simulink model "sensorMCUSlugsMKII"  (Simulink 6.6)
settings: Solver=FixedStepDiscrete  StartTime=0.0  StopTime=10.0  FixedStep=0.01  RelTol=1e-3
InitFcn:
  | mcuInit
values from neighbouring files (symbols this model uses):
  T = 0.01    [initGPS.m]    (also in mcuInit.m)
undefined symbols (not defined in the file or in its folder): baroMeanTemp, baroOffset, baroScale, baroTempK, baseHeight, baseTemp, cubeAccelGain, cubeGyroGain, gaind, getCubeData, getGpsMainData, getMag, hil_getEuler, hil_getRates, hil_getRawRead, hil_getVned, hil_getXYZ, hilRead, lapseRate, logData, magMeanTemp, magOffset, magScale, magTempK, pitotOffset, pitotScale, polesd, powerOffset, powerScale, protParseDecode, sensorMCUInit, spiSend, tempOffset, tempScale, u1, u2, updateAirData, updateAttitude, updateBias, updateDiagnosticFl, updateDiagnosticSh, updateLoadData, updatePilotConsole, updatePosition, updateRawADCData, updateTimeStamp, y1, zerosd
libraries: dsPICdrivers x37, simulink x3, aerolibconvert2 x1
(part 1 of 2)
settings Model: Creator=ASL_Lab  LastModifiedBy=Administrator  BufferReuse=off  ProdHWDeviceType=16-bit Generic
settings OptimizationCC: BlockReduction=off  InlineParams=on  OptimizeBlockIOStorage=off  BufferReuse=off  ExpressionFolding=off  LocalBlockOutputs=off  EfficientFloat2IntCast=on  OptimizeModelRefInitCode=on  LifeSpan=1
settings HardwareCC: ProdBitPerInt=16  ProdEndianess=LittleEndian  ProdWordSize=16  ProdHWDeviceType=16-bit Generic  TargetHWDeviceType=32-bit Generic
settings RTWCC: SystemTargetFile=dspic.tlc  TemplateMakefile=dspic_pic30_gcc.tmf  PostCodeGenCommand=dsPIC_Compile()  Description=Embedded Target for Microchip dsPIC (real-time)  GenerateReport=on  ProcessScript=dspic_make_rtw_hook  CustomHeaderCode="#include \"apDefinitions.h\""  IncludeHyperlinkInReport=on  LaunchReport=on
settings RTWCC: CustomSource=|
  | clib\circBuffer.c
  | clib\sbrk.c
  | clib\gps.c
  | clib\dataLogger.c
  | clib\interProcCommMaster.c
  | clib\conversions.c
  | clib\apUtils.c
  | clib\protDecoder.c
  | clib\DEE.c
  | clib\DEES.s
  | clib\magneto.c
  | clib\adisCube.c
settings CodeAppCC: IgnoreCustomStorageClasses=off
settings STFCustomTargetCC: TargetFcnLib=ansi_tfl_tmw.mat  GenFloatMathFcnCalls=ANSI_C  ModelReferenceCompliant=off  IncludeMdlTerminateFcn=off  CombineOutputUpdateFcns=on  SuppressErrorStatus=on  ERTCustomFileBanners=on  SupportContinuousTime=off  SupportNonInlinedSFcns=off  SystemTargetFile=dspic.tlc
settings ERTTargetCC: TargetFcnLib=ansi_tfl_tmw.mat  GenFloatMathFcnCalls=ANSI_C  ModelReferenceCompliant=off  IncludeMdlTerminateFcn=off  SuppressErrorStatus=on  ModelStepFunctionPrototypeControlCompliant=off  ExtModeMexFile=noextcomm  InlinedParameterPlacement=NonHierarchical  ERTSrcFileBannerTemplate=dsPIC_code_template.cgt  ERTHdrFileBannerTemplate=dsPIC_code_template.cgt  ERTDataSrcFileTemplate=dsPIC_code_template.cgt  ERTDataHdrFileTemplate=dsPIC_code_template.cgt  ERTCustomFileTemplate=dsPIC_main.tlc
settings CustomProperty: DataType=string  Value=C:\PROGRA~1\MATLAB\R2007a\rtw\bin\win32\gmake

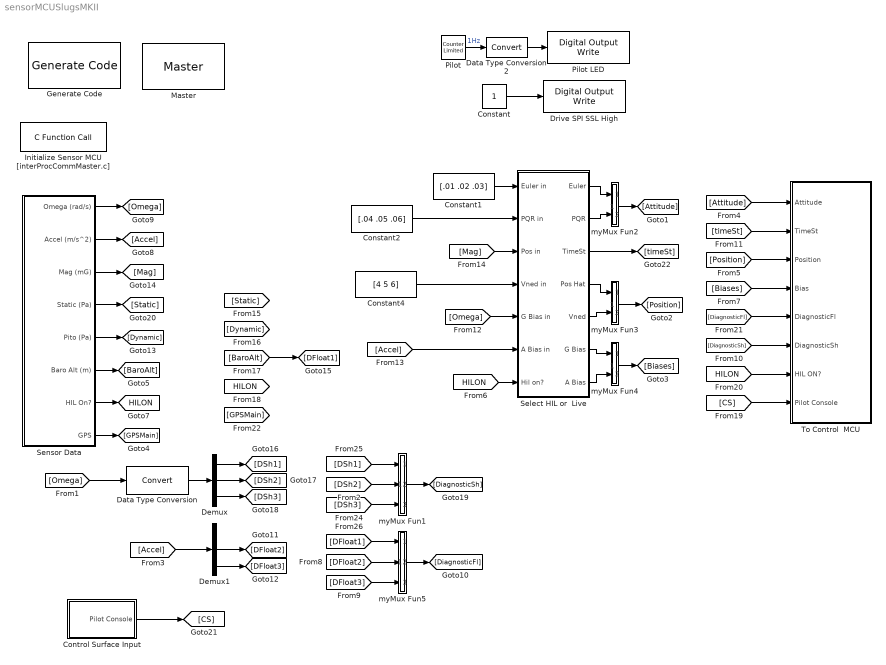
== system sensorMCUSlugsMKII ==
  Constant : Constant  OutDataTypeMode=boolean
  Constant1 : Constant  Value=[.01 .02 .03]  OutDataTypeMode=single
  Constant2 : Constant  Value=[.04 .05 .06]  OutDataTypeMode=single
  Constant4 : Constant  Value=[4 5 6]  OutDataTypeMode=single
  Control Surface Input : Subsystem
  Data Type Conversion : DataTypeConversion  OutDataTypeMode=int16
  Data Type Conversion2 : DataTypeConversion  OutDataTypeMode=boolean
  Demux : Demux  Outputs=3
  Demux1 : Demux  Outputs=3
  Drive SPI SSL High : dsPICdrivers/Digital I//O/Digital Output Write  Tag=dsPIC_Digital_Output  Priority=5  PORT=B  Pin=[ 2]  Simultaneous=off  OrderingInOutPopup=None
  Generate Code : dsPICdrivers/Simulink Configuration/Generate Code
  Initialize Sensor MCU [interProcCommMaster.c] : dsPICdrivers/OTHERS/C Function Call  Tag=dsPIC_dsPIC_CFunctionCall  fctName='sensorMCUInit'  INPUT_SIZE=1  INPUT1=--  INPUT2=--  INPUT3=--  OUTPUT_SIZE=1  OUTPUT1=--  SampleTime=inf  InputType=[ ]  OutputType=[ ]  FctDeclaration=extern void sensorMCUInit();  FctCall=sensorMCUInit();  OrderingInOutPopup=None
  Master : dsPICdrivers/Master  Tag=dsPIC_MASTER  Priority=1  TimeStepType=Timer1  picType=33fJ256MC710  fcy=40000000  Quartz_33f=12e6  PLLActive_33f=on  fcyDesired_33f=40e6  tmr1="[8  49999  0]"  tmr1Info="Time Step : 0.01  ;   Error : 0%  PR1=49999"  tmr2345="[8  0  0  0  0  0  0  0]"  tmr2345cfg=[-1 -1 -1 -1 -1 -1 -1 -1]  IOautoConf=on  typePort="[ 0   0   0   0   0   0   0   0   0   0   0   0   0   0   9   0  10  10  10   0   0   0  10   0   8   8   8   8   0   0   0   0   0   0   0   0   0   0   0   0   0   0   0   0   0   0   0   0   0   0   9   0   0   0   0   0   0   6   6   6   6   0   0   6   0   0   0   0   0   0   0   0   0   0   0   0   0   0   0   0   0   0   0   0   0   0   0   0   0   0   0   0   0   0   0   0   0   0   0   0   0   0   0   0   0   0   0   0   0   0   0   0 ]"  TRIS="[ 65535  65464  65535  65535  65535  65535  65535 ]"  ADPCFG=71  MasterBusyPort=B1  MasterOverloadPort=B6  FOSC=External Clock  ClockSwitchMonitor=Both disabled  TempProtection_33f=TEMP_ON  FPBOR=<empty>  PWRT=64ms  MCLR=<empty>  PowerSave=off  OverrideFcy=off  NewFcy=1e6  PR2345="[65535  65535  65535  65535  65535  65535  65535  65535]"
  Pilot : simulink/Sources/Counter Limited  SystemSampleTime=-1  uplimit=1  tsamp=1.0
  Pilot LED : dsPICdrivers/Digital I//O/Digital Output Write  Tag=dsPIC_Digital_Output  Priority=5  PORT=B  Pin=[0]  Simultaneous=off  OrderingInOutPopup=None
  Select HIL or  Live : Subsystem
  Sensor Data : Subsystem
  To Control  MCU : Subsystem
  myMux Fun1 : Stateflow chart
  myMux Fun2 : Stateflow chart
  myMux Fun3 : Stateflow chart
  myMux Fun4 : Stateflow chart
  myMux Fun5 : Stateflow chart
  tag scope: HILON=global
  wires:
  Pilot/1 -> Data Type Conversion2/1  "1Hz"
  Data Type Conversion2/1 -> Pilot LED/1
  Constant/1 -> Drive SPI SSL High/1
  myMux Fun2/1(y) -> [Attitude]
  myMux Fun3/1(y) -> [Position]
  myMux Fun4/1(y) -> [Biases]
  Demux/1 -> [DSh1]
  Demux/2 -> [DSh2]
  Demux/3 -> [DSh3]
  Control Surface Input/1(Pilot Console) -> [CS]
  [Position] -> To Control  MCU/3(Position)
  [Biases] -> To Control  MCU/4(Bias)
  [DiagnosticFl] -> To Control  MCU/5(DiagnosticFl)
  [HILON] -> To Control  MCU/7(HIL ON?)
  [CS] -> To Control  MCU/8(Pilot Console)
  [Attitude] -> To Control  MCU/1(Attitude)
  Select HIL or  Live/1(Euler) -> myMux Fun2/1(u1)
  Select HIL or  Live/2(PQR) -> myMux Fun2/2(u2)
  Select HIL or  Live/3(TimeSt) -> [timeSt]
  Select HIL or  Live/4(Pos Hat) -> myMux Fun3/1(u1)
  Select HIL or  Live/5(Vned) -> myMux Fun3/2(u2)
  Select HIL or  Live/6(G Bias) -> myMux Fun4/1(u1)
  Select HIL or  Live/7(A Bias) -> myMux Fun4/2(u2)
  [DSh1] -> myMux Fun1/1(u1)
  [DSh2] -> myMux Fun1/2(u2)
  [DSh3] -> myMux Fun1/3(u3)
  [DFloat1] -> myMux Fun5/1(u1)
  [DFloat2] -> myMux Fun5/2(u2)
  [DFloat3] -> myMux Fun5/3(u3)
  myMux Fun1/1(y) -> [DiagnosticSh]
  myMux Fun5/1(y) -> [DiagnosticFl]
  [DiagnosticSh] -> To Control  MCU/6(DiagnosticSh)
  [timeSt] -> To Control  MCU/2(TimeSt)
  Sensor Data/2(Accel (m/s^2)) -> [Accel]
  Sensor Data/1(Omega (rad/s)) -> [Omega]
  Sensor Data/3(Mag (mG)) -> [Mag]
  Sensor Data/4(Static (Pa)) -> [Static]
  Sensor Data/5(Pito (Pa)) -> [Dynamic]
  Sensor Data/6(Baro Alt (m)) -> [BaroAlt]
  Sensor Data/7(HIL On?) -> [HILON]
  Sensor Data/8(GPS) -> [GPSMain]
  Demux1/2 -> [DFloat2]
  Demux1/3 -> [DFloat3]
  Data Type Conversion/1 -> Demux/1
  [Omega] -> Data Type Conversion/1
  [Accel] -> Demux1/1
  [HILON] -> Select HIL or  Live/7(Hil on?)
  Constant1/1 -> Select HIL or  Live/1(Euler in)
  Constant2/1 -> Select HIL or  Live/2(PQR in)
  [Mag] -> Select HIL or  Live/3(Pos in)
  Constant4/1 -> Select HIL or  Live/4(Vned in)
  [Omega] -> Select HIL or  Live/5(G Bias in)
  [Accel] -> Select HIL or  Live/6(A Bias in)
  [BaroAlt] -> [DFloat1]

== system sensorMCUSlugsMKII/Control Surface Input ==
  Input Capture : dsPICdrivers/Peripheral I//O/Input Capture  Tag=dsPIC_PWM_IC  Priority=5  IntPriority=6  Channel=[ 2 3 4 5 8]  Channel_UP_Down_Periode="[1  1  1  1  1]"  MaxChannel="[0.0025      0.0025      0.0025      0.0025      0.0025]"  SafeMarge="[10  10  10  10  10]"  MaxName=' IC2max , IC3max , IC4max , IC5max , IC8max '  Precision="[13.7469      13.7469      13.7469      13.7469      13.7469]"  Timer="[2  2  2  2  2]"  ChangeDetected="[0  0  0  0  0]"  ChangeDetectedPortRef=3  SampleTime=.01  Status=OK
  myMux Fun5 : Stateflow chart
  Pilot Console : Outport
  wires:
  myMux Fun5/1(y) -> Pilot Console/1
  Input Capture/1 -> myMux Fun5/1(u1)
  Input Capture/2 -> myMux Fun5/2(u2)
  Input Capture/3 -> myMux Fun5/3(u3)
  Input Capture/4 -> myMux Fun5/4(u4)
  Input Capture/5 -> myMux Fun5/5(u5)

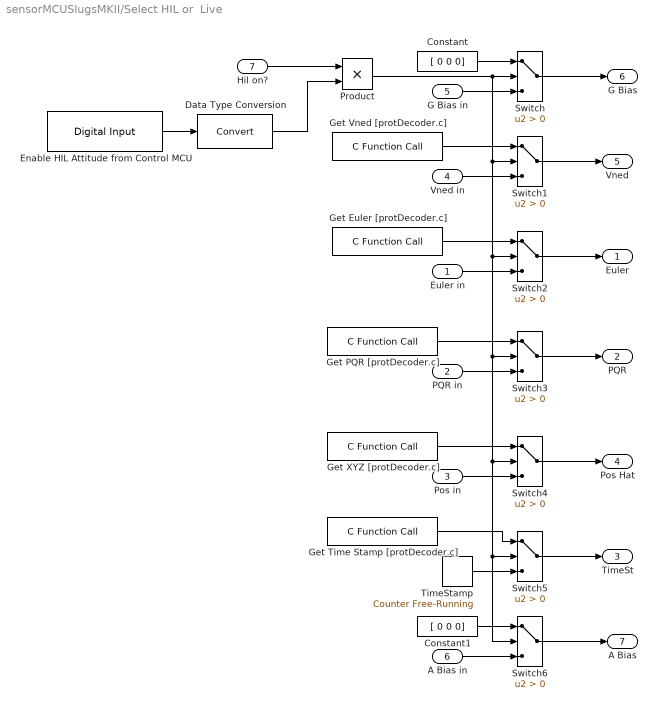
== system sensorMCUSlugsMKII/Select HIL or  Live ==
  Euler in : Inport
  PQR in : Inport  Port=2
  Pos in : Inport  Port=3
  Vned in : Inport  Port=4
  G Bias in : Inport  Port=5
  A Bias in : Inport  Port=6
  Hil on? : Inport  Port=7
  Constant : Constant  Value=[ 0 0 0]  OutDataTypeMode=single
  Constant1 : Constant  Value=[ 0 0 0]  OutDataTypeMode=single
  Data Type Conversion : DataTypeConversion  OutDataTypeMode=uint8
  Enable HIL Attitude from Control MCU : dsPICdrivers/Digital I//O/Digital Input  Tag=dsPIC_Digital_Input  PORT=A  Pin=[14]  SampleTime=.01  OrderingInOutPopup=None
  Get Euler [protDecoder.c] : dsPICdrivers/OTHERS/C Function Call  Tag=dsPIC_dsPIC_CFunctionCall  fctName='hil_getEuler'  INPUT_SIZE=1  INPUT1=--  INPUT2=--  INPUT3=--  OUTPUT_SIZE=3  OUTPUT1=real32  SampleTime=.01  InputType=[ ]  OutputType=[ 7 ]  FctDeclaration=extern void hil_getEuler(real32_T* y1);  FctCall=hil_getEuler(*%y1);  OrderingInOutPopup=None
  Get PQR [protDecoder.c] : dsPICdrivers/OTHERS/C Function Call  Tag=dsPIC_dsPIC_CFunctionCall  fctName='hil_getRates'  INPUT_SIZE=1  INPUT1=--  INPUT2=--  INPUT3=--  OUTPUT_SIZE=3  OUTPUT1=real32  SampleTime=.01  InputType=[ ]  OutputType=[ 7 ]  FctDeclaration=extern void hil_getRates(real32_T* y1);  FctCall=hil_getRates(*%y1);  OrderingInOutPopup=None
  Get Time Stamp [protDecoder.c] : dsPICdrivers/OTHERS/C Function Call  Tag=dsPIC_dsPIC_CFunctionCall  fctName='hil_getTs'  INPUT_SIZE=1  INPUT1=--  INPUT2=--  INPUT3=--  OUTPUT_SIZE=1  OUTPUT1=uint16  SampleTime=.01  InputType=[ ]  OutputType=[ 4 ]  FctDeclaration=extern uint16_T hil_getTs();  FctCall=%y1 = hil_getTs();  OrderingInOutPopup=None
  Get Vned [protDecoder.c] : dsPICdrivers/OTHERS/C Function Call  Tag=dsPIC_dsPIC_CFunctionCall  fctName='hil_getVned'  INPUT_SIZE=1  INPUT1=--  INPUT2=--  INPUT3=--  OUTPUT_SIZE=3  OUTPUT1=real32  SampleTime=.01  InputType=[ ]  OutputType=[ 7 ]  FctDeclaration=extern void hil_getVned(real32_T* y1);  FctCall=hil_getVned(*%y1);  OrderingInOutPopup=None
  Get XYZ [protDecoder.c] : dsPICdrivers/OTHERS/C Function Call  Tag=dsPIC_dsPIC_CFunctionCall  fctName='hil_getXYZ'  INPUT_SIZE=1  INPUT1=--  INPUT2=--  INPUT3=--  OUTPUT_SIZE=3  OUTPUT1=real32  SampleTime=.01  InputType=[ ]  OutputType=[ 7 ]  FctDeclaration=extern void hil_getXYZ(real32_T* y1);  FctCall=hil_getXYZ(*%y1);  OrderingInOutPopup=None
  Product : Product  OutDataTypeMode=uint8  RndMeth=Zero
  Switch{,1..6} (7 alike) : Switch  Criteria=u2 > Threshold
  TimeStamp : simulink/Sources/Counter Free-Running  SystemSampleTime=-1  NumBits=16  tsamp=.01
  Euler : Outport
  PQR : Outport  Port=2
  TimeSt : Outport  Port=3
  Pos Hat : Outport  Port=4
  Vned : Outport  Port=5
  G Bias : Outport  Port=6
  A Bias : Outport  Port=7
  wires:
  Switch/1 -> G Bias/1
  Constant/1 -> Switch/1
  Product/1 -> Switch/2, Switch1/2, Switch2/2, Switch3/2, Switch4/2, Switch5/2, Switch6/2
  G Bias in/1 -> Switch/3
  Switch1/1 -> Vned/1
  Get Vned [protDecoder.c]/1 -> Switch1/1
  Vned in/1 -> Switch1/3
  Get Euler [protDecoder.c]/1 -> Switch2/1
  Euler in/1 -> Switch2/3
  Switch2/1 -> Euler/1
  Get PQR [protDecoder.c]/1 -> Switch3/1
  PQR in/1 -> Switch3/3
  Switch3/1 -> PQR/1
  Get XYZ [protDecoder.c]/1 -> Switch4/1
  Pos in/1 -> Switch4/3
  Switch4/1 -> Pos Hat/1
  TimeStamp/1 -> Switch5/3
  Get Time Stamp [protDecoder.c]/1 -> Switch5/1
  Enable HIL Attitude from Control MCU/1 -> Data Type Conversion/1
  Hil on?/1 -> Product/1
  Data Type Conversion/1 -> Product/2
  Switch5/1 -> TimeSt/1
  Switch6/1 -> A Bias/1
  Constant1/1 -> Switch6/1
  A Bias in/1 -> Switch6/3

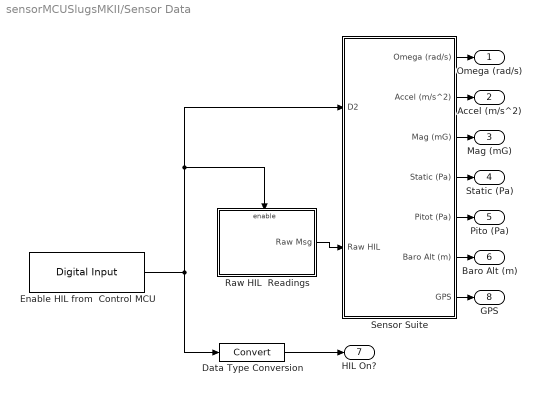
== system sensorMCUSlugsMKII/Sensor Data ==
  Data Type Conversion : DataTypeConversion  OutDataTypeMode=uint8  SampleTime=0.01
  Enable HIL from  Control MCU : dsPICdrivers/Digital I//O/Digital Input  Tag=dsPIC_Digital_Input  PORT=D  Pin=[2]  SampleTime=.01  OrderingInOutPopup=None
  Raw HIL  Readings : Subsystem
  Sensor Suite : Subsystem
  Omega (rad/s) : Outport
  Accel (m/s^2) : Outport  Port=2
  Mag (mG) : Outport  Port=3
  Static (Pa) : Outport  Port=4
  Pito (Pa) : Outport  Port=5
  Baro Alt (m) : Outport  Port=6
  HIL On? : Outport  Port=7
  GPS : Outport  Port=8
  wires:
  Raw HIL  Readings/1(Raw Msg) -> Sensor Suite/2(Raw HIL)
  Enable HIL from  Control MCU/1 -> Raw HIL  Readings/Enable, Sensor Suite/1(D2), Data Type Conversion/1
  Data Type Conversion/1 -> HIL On?/1
  Sensor Suite/1(Omega (rad/s)) -> Omega (rad/s)/1
  Sensor Suite/2(Accel (m/s^2)) -> Accel (m/s^2)/1
  Sensor Suite/3(Mag (mG)) -> Mag (mG)/1
  Sensor Suite/4(Static (Pa)) -> Static (Pa)/1
  Sensor Suite/5(Pitot (Pa)) -> Pito (Pa)/1
  Sensor Suite/6(Baro Alt (m)) -> Baro Alt (m)/1
  Sensor Suite/7(GPS) -> GPS/1

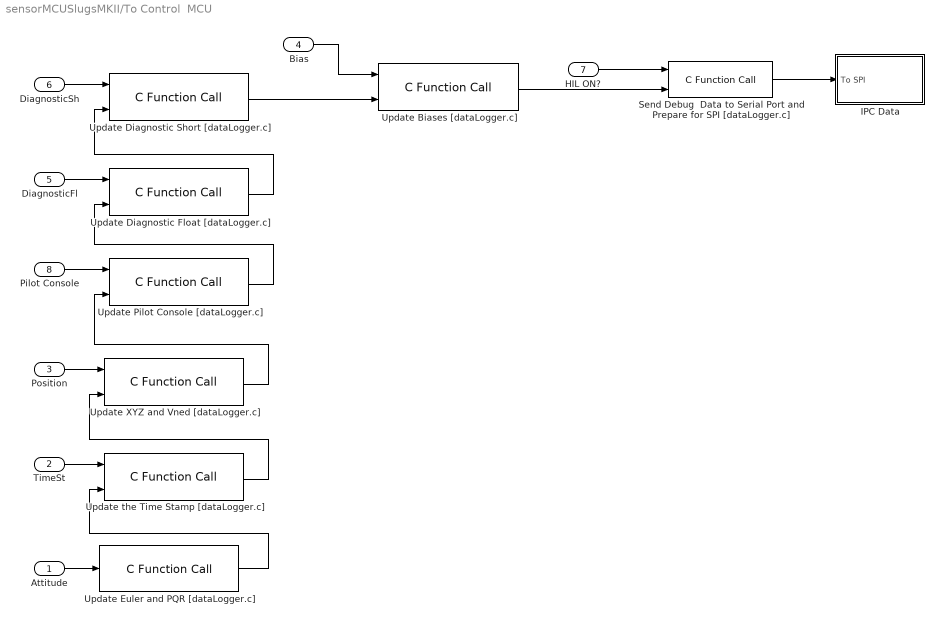
== system sensorMCUSlugsMKII/To Control  MCU ==
  Attitude : Inport
  TimeSt : Inport  Port=2
  Position : Inport  Port=3
  Bias : Inport  Port=4
  DiagnosticFl : Inport  Port=5
  DiagnosticSh : Inport  Port=6
  HIL ON? : Inport  Port=7
  Pilot Console : Inport  Port=8
  IPC Data : Subsystem
  Send Debug  Data to Serial Port and Prepare for SPI [dataLogger.c] : dsPICdrivers/OTHERS/C Function Call  Tag=dsPIC_dsPIC_CFunctionCall  fctName='logData'  INPUT_SIZE=1  INPUT1=uint8  INPUT2=--  INPUT3=--  OUTPUT_SIZE=104  OUTPUT1=uint8  SampleTime=-1  InputType=[ 2 ]  OutputType=[ 2 ]  FctDeclaration=extern void logData(uint8_T u1,uint8_T* y1);  FctCall=logData(%u1, *%y1);  OrderingInOutPopup=Input
  Update Biases [dataLogger.c] : dsPICdrivers/OTHERS/C Function Call  Tag=dsPIC_dsPIC_CFunctionCall  fctName='updateBias'  INPUT_SIZE=6  INPUT1=real32  INPUT2=--  INPUT3=--  OUTPUT_SIZE=1  OUTPUT1=--  SampleTime=.01  InputType=[ 7 ]  OutputType=[ ]  FctDeclaration=extern void updateBias(real32_T* u1);  FctCall=updateBias(*%u1);  OrderingInOutPopup=Input & Output
  Update Diagnostic Float [dataLogger.c] : dsPICdrivers/OTHERS/C Function Call  Tag=dsPIC_dsPIC_CFunctionCall  fctName='updateDiagnosticFl'  INPUT_SIZE=3  INPUT1=real32  INPUT2=--  INPUT3=--  OUTPUT_SIZE=1  OUTPUT1=--  SampleTime=.01  InputType=[ 7 ]  OutputType=[ ]  FctDeclaration=extern void updateDiagnosticFl(real32_T* u1);  FctCall=updateDiagnosticFl(*%u1);  OrderingInOutPopup=Input & Output
  Update Diagnostic Short [dataLogger.c] : dsPICdrivers/OTHERS/C Function Call  Tag=dsPIC_dsPIC_CFunctionCall  fctName='updateDiagnosticSh'  INPUT_SIZE=3  INPUT1=int16  INPUT2=--  INPUT3=--  OUTPUT_SIZE=1  OUTPUT1=--  SampleTime=.01  InputType=[ 3 ]  OutputType=[ ]  FctDeclaration=extern void updateDiagnosticSh(int16_T* u1);  FctCall=updateDiagnosticSh(*%u1);  OrderingInOutPopup=Input & Output
  Update Euler and PQR [dataLogger.c] : dsPICdrivers/OTHERS/C Function Call  Tag=dsPIC_dsPIC_CFunctionCall  fctName='updateAttitude'  INPUT_SIZE=6  INPUT1=real32  INPUT2=--  INPUT3=--  OUTPUT_SIZE=1  OUTPUT1=--  SampleTime=.01  InputType=[ 7 ]  OutputType=[ ]  FctDeclaration=extern void updateAttitude(real32_T* u1);  FctCall=updateAttitude(*%u1);  OrderingInOutPopup=Output
  Update Pilot Console [dataLogger.c] : dsPICdrivers/OTHERS/C Function Call  Tag=dsPIC_dsPIC_CFunctionCall  fctName='updatePilotConsole'  INPUT_SIZE=5  INPUT1=uint16  INPUT2=--  INPUT3=--  OUTPUT_SIZE=1  OUTPUT1=--  SampleTime=.01  InputType=[ 4 ]  OutputType=[ ]  FctDeclaration=extern void updatePilotConsole(uint16_T* u1);  FctCall=updatePilotConsole(*%u1);  OrderingInOutPopup=Input & Output
  Update XYZ and Vned [dataLogger.c] : dsPICdrivers/OTHERS/C Function Call  Tag=dsPIC_dsPIC_CFunctionCall  fctName='updatePosition'  INPUT_SIZE=6  INPUT1=real32  INPUT2=--  INPUT3=--  OUTPUT_SIZE=1  OUTPUT1=--  SampleTime=.01  InputType=[ 7 ]  OutputType=[ ]  FctDeclaration=extern void updatePosition(real32_T* u1);  FctCall=updatePosition(*%u1);  OrderingInOutPopup=Input & Output
  Update the Time Stamp [dataLogger.c] : dsPICdrivers/OTHERS/C Function Call  Tag=dsPIC_dsPIC_CFunctionCall  fctName='updateTimeStamp'  INPUT_SIZE=1  INPUT1=uint16  INPUT2=--  INPUT3=--  OUTPUT_SIZE=1  OUTPUT1=--  SampleTime=.01  InputType=[ 4 ]  OutputType=[ ]  FctDeclaration=extern void updateTimeStamp(uint16_T u1);  FctCall=updateTimeStamp(%u1);  OrderingInOutPopup=Input & Output
  wires:
  Send Debug  Data to Serial Port and Prepare for SPI [dataLogger.c]/1 -> IPC Data/1(To SPI)
  HIL ON?/1 -> Send Debug  Data to Serial Port and Prepare for SPI [dataLogger.c]/1
  Attitude/1 -> Update Euler and PQR [dataLogger.c]/1
  Update Euler and PQR [dataLogger.c]/1 -> Update the Time Stamp [dataLogger.c]/2
  TimeSt/1 -> Update the Time Stamp [dataLogger.c]/1
  Update the Time Stamp [dataLogger.c]/1 -> Update XYZ and Vned [dataLogger.c]/2
  Position/1 -> Update XYZ and Vned [dataLogger.c]/1
  Update XYZ and Vned [dataLogger.c]/1 -> Update Pilot Console [dataLogger.c]/2
  Pilot Console/1 -> Update Pilot Console [dataLogger.c]/1
  DiagnosticFl/1 -> Update Diagnostic Float [dataLogger.c]/1
  Update Pilot Console [dataLogger.c]/1 -> Update Diagnostic Float [dataLogger.c]/2
  Update Diagnostic Float [dataLogger.c]/1 -> Update Diagnostic Short [dataLogger.c]/2
  DiagnosticSh/1 -> Update Diagnostic Short [dataLogger.c]/1
  Update Biases [dataLogger.c]/1 -> Send Debug  Data to Serial Port and Prepare for SPI [dataLogger.c]/2
  Update Diagnostic Short [dataLogger.c]/1 -> Update Biases [dataLogger.c]/2
  Bias/1 -> Update Biases [dataLogger.c]/1

== system sensorMCUSlugsMKII/Sensor Data/Raw HIL  Readings ==
  Enable : EnablePort
  GetRawMsg [protDecoder.c] : dsPICdrivers/OTHERS/C Function Call  Tag=dsPIC_dsPIC_CFunctionCall  fctName='hil_getRawRead'  INPUT_SIZE=1  INPUT1=--  INPUT2=--  INPUT3=--  OUTPUT_SIZE=13  OUTPUT1=int16  SampleTime=0.01  InputType=[ ]  OutputType=[ 3 ]  FctDeclaration=extern void hil_getRawRead(int16_T* y1);  FctCall=hil_getRawRead(*%y1);  OrderingInOutPopup=Input
  Parser/Decoder [protDecoder.c] : dsPICdrivers/OTHERS/C Function Call  Tag=dsPIC_dsPIC_CFunctionCall  fctName='protParseDecode'  INPUT_SIZE=103  INPUT1=uint8  INPUT2=--  INPUT3=--  OUTPUT_SIZE=1  OUTPUT1=--  SampleTime=-1  InputType=[ 2 ]  OutputType=[ ]  FctDeclaration=extern void protParseDecode(uint8_T* u1);  FctCall=protParseDecode(*%u1);  OrderingInOutPopup=Output
  Read Data from HIL3 [dataLogger.c] : dsPICdrivers/OTHERS/C Function Call  Tag=dsPIC_dsPIC_CFunctionCall  fctName='hilRead'  INPUT_SIZE=1  INPUT1=--  INPUT2=--  INPUT3=--  OUTPUT_SIZE=103  OUTPUT1=uint8  SampleTime=0.01  InputType=[ ]  OutputType=[ 2 ]  FctDeclaration=extern void hilRead(uint8_T* y1);  FctCall=hilRead(*%y1);  OrderingInOutPopup=None
  Raw Msg : Outport
  wires:
  GetRawMsg [protDecoder.c]/1 -> Raw Msg/1
  Read Data from HIL3 [dataLogger.c]/1 -> Parser/Decoder [protDecoder.c]/1
  Parser/Decoder [protDecoder.c]/1 -> GetRawMsg [protDecoder.c]/1

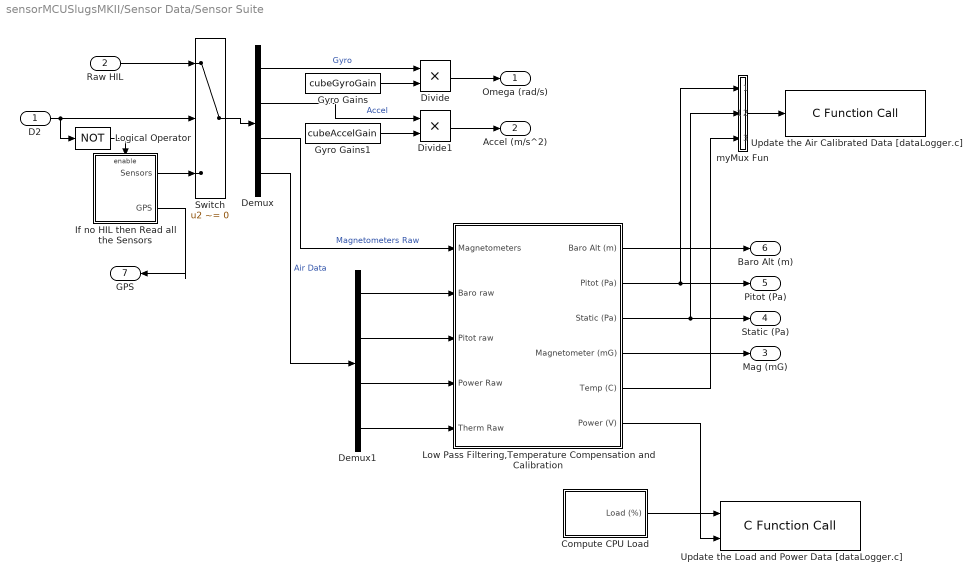
== system sensorMCUSlugsMKII/Sensor Data/Sensor Suite ==
  D2 : Inport
  Raw HIL : Inport  Port=2
  Compute CPU Load : Subsystem
  Demux : Demux  Outputs=[3 3 3 4]
  Demux1 : Demux
  Divide : Product  OutDataTypeMode=single  OutScaling=2^-10
  Divide1 : Product  OutDataTypeMode=single  OutScaling=2^-10
  Gyro Gains : Constant  Value=cubeGyroGain  OutDataTypeMode=single
  Gyro Gains1 : Constant  Value=cubeAccelGain  OutDataTypeMode=single
  If no HIL then Read all the Sensors : Subsystem
  Logical Operator : Logic  Operator=NOT  AllPortsSameDT=off  OutDataTypeMode=Boolean
  Low Pass Filtering,Temperature Compensation and Calibration : Subsystem
  Switch : Switch  Criteria=u2 ~= 0  SampleTime=0.01
  Update the Air Calibrated Data [dataLogger.c] : dsPICdrivers/OTHERS/C Function Call  Tag=dsPIC_dsPIC_CFunctionCall  fctName='updateAirData'  INPUT_SIZE=3  INPUT1=real32  INPUT2=--  INPUT3=--  OUTPUT_SIZE=1  OUTPUT1=--  SampleTime=.01  InputType=[ 7 ]  OutputType=[ ]  FctDeclaration=extern void updateAirData(real32_T* u1);  FctCall=updateAirData(*%u1);  OrderingInOutPopup=None
  Update the Load and Power Data [dataLogger.c] : dsPICdrivers/OTHERS/C Function Call  Tag=dsPIC_dsPIC_CFunctionCall  fctName='updateLoadData'  INPUT_SIZE=1  INPUT1=uint8  INPUT2=uint16  INPUT3=--  OUTPUT_SIZE=1  OUTPUT1=--  SampleTime=.01  InputType=[ 2 4 ]  OutputType=[ ]  FctDeclaration=extern void updateLoadData(uint8_T u1, uint16_T u2);  FctCall=updateLoadData(%u1, %u2);  OrderingInOutPopup=None
  myMux Fun : Stateflow chart
  Omega (rad/s) : Outport
  Accel (m/s^2) : Outport  Port=2
  Mag (mG) : Outport  Port=3
  Static (Pa) : Outport  Port=4
  Pitot (Pa) : Outport  Port=5
  Baro Alt (m) : Outport  Port=6
  GPS : Outport  Orientation=left  Port=7
  wires:
  Switch/1 -> Demux/1
  D2/1 -> Switch/2, Logical Operator/1
  If no HIL then Read all the Sensors/1(Sensors) -> Switch/3
  Logical Operator/1 -> If no HIL then Read all the Sensors/Enable
  Raw HIL/1 -> Switch/1
  Low Pass Filtering,Temperature Compensation and Calibration/1(Baro Alt (m)) -> Baro Alt (m)/1
  Gyro Gains/1 -> Divide/2
  Demux/1 -> Divide/1  "Gyro"
  Divide/1 -> Omega (rad/s)/1
  Gyro Gains1/1 -> Divide1/2
  Demux/2 -> Divide1/1  "Accel"
  Divide1/1 -> Accel (m/s^2)/1
  Demux/4 -> Demux1/1  "Air Data"
  Demux1/1 -> Low Pass Filtering,Temperature Compensation and Calibration/2(Baro raw)
  Demux1/2 -> Low Pass Filtering,Temperature Compensation and Calibration/3(Pitot raw)
  Demux1/4 -> Low Pass Filtering,Temperature Compensation and Calibration/5(Therm Raw)
  Demux/3 -> Low Pass Filtering,Temperature Compensation and Calibration/1(Magnetometers)  "Magnetometers Raw"
  Demux1/3 -> Low Pass Filtering,Temperature Compensation and Calibration/4(Power Raw)
  Low Pass Filtering,Temperature Compensation and Calibration/2(Pitot (Pa)) -> Pitot (Pa)/1, myMux Fun/1(u1)
  Low Pass Filtering,Temperature Compensation and Calibration/3(Static (Pa)) -> Static (Pa)/1, myMux Fun/2(u2)
  Low Pass Filtering,Temperature Compensation and Calibration/4(Magnetometer (mG)) -> Mag (mG)/1
  myMux Fun/1(y) -> Update the Air Calibrated Data [dataLogger.c]/1
  Low Pass Filtering,Temperature Compensation and Calibration/5(Temp (C)) -> myMux Fun/3(u3)
  Compute CPU Load/1(Load (%)) -> Update the Load and Power Data [dataLogger.c]/1
  Low Pass Filtering,Temperature Compensation and Calibration/6(Power (V)) -> Update the Load and Power Data [dataLogger.c]/2
  If no HIL then Read all the Sensors/2(GPS) -> GPS/1

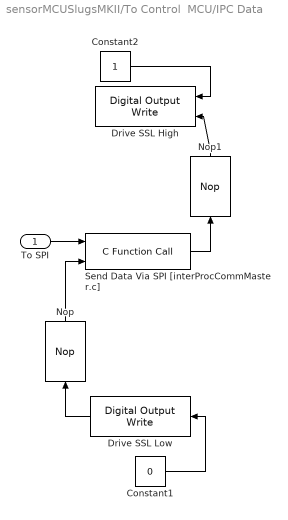
== system sensorMCUSlugsMKII/To Control  MCU/IPC Data ==
  To SPI : Inport
  Constant1 : Constant  Value=0  OutDataTypeMode=boolean  SampleTime=.01
  Constant2 : Constant  OutDataTypeMode=boolean
  Drive SSL High : dsPICdrivers/Digital I//O/Digital Output Write  Tag=dsPIC_Digital_Output  Orientation=left  Priority=5  PORT=B  Pin=[ 2]  Simultaneous=off  OrderingInOutPopup=Input
  Drive SSL Low : dsPICdrivers/Digital I//O/Digital Output Write  Tag=dsPIC_Digital_Output  Orientation=left  Priority=5  PORT=B  Pin=[ 2]  Simultaneous=off  OrderingInOutPopup=Output
  Nop : dsPICdrivers/OTHERS/Nop  Tag=dsPIC_Reset  Orientation=up  NbrNop=10
  Nop1 : dsPICdrivers/OTHERS/Nop  Tag=dsPIC_Reset  Orientation=up  NbrNop=10
  Send Data Via SPI [interProcCommMaster.c] : dsPICdrivers/OTHERS/C Function Call  Tag=dsPIC_dsPIC_CFunctionCall  fctName='spiSend'  INPUT_SIZE=104  INPUT1=uint8  INPUT2=--  INPUT3=--  OUTPUT_SIZE=1  OUTPUT1=--  SampleTime=-1  InputType=[ 2 ]  OutputType=[ ]  FctDeclaration=extern void spiSend(uint8_T* u1);  FctCall=spiSend(*%u1);  OrderingInOutPopup=Input & Output
  wires:
  Constant1/1 -> Drive SSL Low/1
  Drive SSL Low/1 -> Nop/1
  Constant2/1 -> Drive SSL High/1
  Send Data Via SPI [interProcCommMaster.c]/1 -> Nop1/1
  To SPI/1 -> Send Data Via SPI [interProcCommMaster.c]/1
  Nop/1 -> Send Data Via SPI [interProcCommMaster.c]/2
  Nop1/1 -> Drive SSL High/2

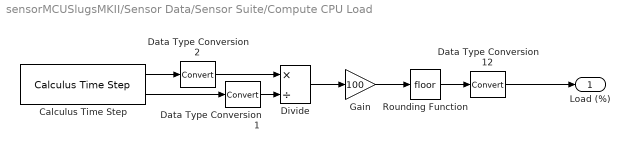
== system sensorMCUSlugsMKII/Sensor Data/Sensor Suite/Compute CPU Load ==
  Calculus Time Step : dsPICdrivers/OTHERS/Calculus Time Step  Tag=dsPIC_CalculusTimeStep  SampleTime=0.01  PR1chk=on
  Data Type Conversion1 : DataTypeConversion  OutDataTypeMode=single
  Data Type Conversion12 : DataTypeConversion  OutDataTypeMode=uint8
  Data Type Conversion2 : DataTypeConversion  OutDataTypeMode=single
  Divide : Product  Inputs=*/  OutDataTypeMode=double  OutScaling=2^-10
  Gain : Gain  Gain=100
  Rounding Function : Rounding
  Load (%) : Outport
  wires:
  Calculus Time Step/1 -> Data Type Conversion2/1
  Calculus Time Step/2 -> Data Type Conversion1/1
  Divide/1 -> Gain/1
  Rounding Function/1 -> Data Type Conversion12/1
  Data Type Conversion1/1 -> Divide/2
  Data Type Conversion2/1 -> Divide/1
  Data Type Conversion12/1 -> Load (%)/1
  Gain/1 -> Rounding Function/1

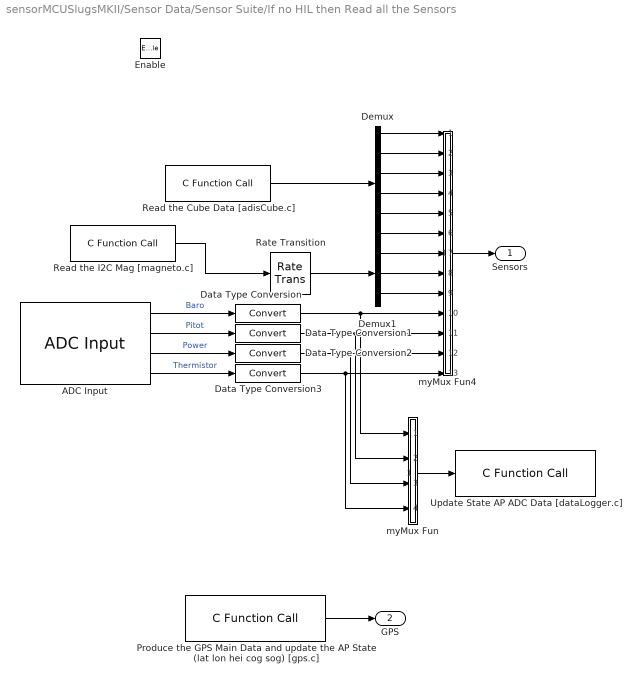
== system sensorMCUSlugsMKII/Sensor Data/Sensor Suite/If no HIL then Read all the Sensors ==
  Enable : EnablePort
  ADC Input : dsPICdrivers/Peripheral I//O/ADC Input  Tag=dsPIC_ADC  Priority=5  ADC_TYPE=12 bits  ADC_MODE=Continuous sampling & get last channel value  NbrSampleStep=1  VoltRefpopup="AVdd  -  AVss"  OutFormatBitspopup=0000 dddd dddd dddd : Integer  InterruptPriority=6  ANCHANNELS=[8 9 10 11]  MaxName=ANmax = 4095  Rin=200  ADCS=53  SAMC=1  Temperature=25  DMAChannel=1  SampleTime=.01  Status="OK  |  Tsmp=6.750e-007 |  T/Channel=1.012e-005 |  Tall=4.050e-005"  SSRC=auto convert
  Data Type Conversion{,1..3} (4 alike) : DataTypeConversion  OutDataTypeMode=int16
  Demux : Demux  Outputs=6
  Demux1 : Demux  Outputs=3
  Produce the GPS Main Data and update the AP State (lat lon hei cog sog) [gps.c] : dsPICdrivers/OTHERS/C Function Call  Tag=dsPIC_dsPIC_CFunctionCall  fctName='getGpsMainData'  INPUT_SIZE=1  INPUT1=--  INPUT2=--  INPUT3=--  OUTPUT_SIZE=5  OUTPUT1=real32  SampleTime=.01  InputType=[ ]  OutputType=[ 7 ]  FctDeclaration=extern void getGpsMainData(real32_T* y1);  FctCall=getGpsMainData(*%y1);  OrderingInOutPopup=None
  Rate Transition : RateTransition  OutPortSampleTime=0.01
  Read the Cube Data [adisCube.c] : dsPICdrivers/OTHERS/C Function Call  Tag=dsPIC_dsPIC_CFunctionCall  fctName='getCubeData'  INPUT_SIZE=1  INPUT1=--  INPUT2=--  INPUT3=--  OUTPUT_SIZE=6  OUTPUT1=int16  SampleTime=.01  InputType=[ ]  OutputType=[ 3 ]  FctDeclaration=extern void getCubeData(int16_T* y1);  FctCall=getCubeData(*%y1);  OrderingInOutPopup=None
  Read the I2C Mag [magneto.c] : dsPICdrivers/OTHERS/C Function Call  Tag=dsPIC_dsPIC_CFunctionCall  fctName='getMag'  INPUT_SIZE=1  INPUT1=--  INPUT2=--  INPUT3=--  OUTPUT_SIZE=3  OUTPUT1=int16  SampleTime=.01  InputType=[ ]  OutputType=[ 3 ]  FctDeclaration=extern void getMag(int16_T* y1);  FctCall=getMag(*%y1);  OrderingInOutPopup=None
  Update State AP ADC Data [dataLogger.c] : dsPICdrivers/OTHERS/C Function Call  Tag=dsPIC_dsPIC_CFunctionCall  fctName='updateRawADCData'  INPUT_SIZE=4  INPUT1=int16  INPUT2=--  INPUT3=--  OUTPUT_SIZE=1  OUTPUT1=--  SampleTime=.01  InputType=[ 3 ]  OutputType=[ ]  FctDeclaration=extern void updateRawADCData(int16_T* u1);  FctCall=updateRawADCData(*%u1);  OrderingInOutPopup=None
  myMux Fun : Stateflow chart
  myMux Fun4 : Stateflow chart
  Sensors : Outport
  GPS : Outport  Port=2
  wires:
  myMux Fun4/1(y) -> Sensors/1
  Read the Cube Data [adisCube.c]/1 -> Demux/1
  Read the I2C Mag [magneto.c]/1 -> Rate Transition/1
  Demux/1 -> myMux Fun4/1(u1)
  Demux/2 -> myMux Fun4/2(u2)
  Demux/3 -> myMux Fun4/3(u3)
  Demux/4 -> myMux Fun4/4(u4)
  Demux/5 -> myMux Fun4/5(u5)
  Demux/6 -> myMux Fun4/6(u6)
  Demux1/1 -> myMux Fun4/7(u7)
  Demux1/2 -> myMux Fun4/8(u8)
  Demux1/3 -> myMux Fun4/9(u9)
  ADC Input/1 -> Data Type Conversion/1  "Baro"
  ADC Input/2 -> Data Type Conversion1/1  "Pitot"
  ADC Input/3 -> Data Type Conversion2/1  "Power"
  ADC Input/4 -> Data Type Conversion3/1  "Thermistor"
  myMux Fun/1(y) -> Update State AP ADC Data [dataLogger.c]/1
  Rate Transition/1 -> Demux1/1
  Data Type Conversion/1 -> myMux Fun4/10(u10), myMux Fun/1(u1)
  Data Type Conversion1/1 -> myMux Fun4/11(u11), myMux Fun/2(u2)
  Data Type Conversion2/1 -> myMux Fun4/12(u12), myMux Fun/3(u3)
  Data Type Conversion3/1 -> myMux Fun4/13(u13), myMux Fun/4(u4)
  Produce the GPS Main Data and update the AP State (lat lon hei cog sog) [gps.c]/1 -> GPS/1

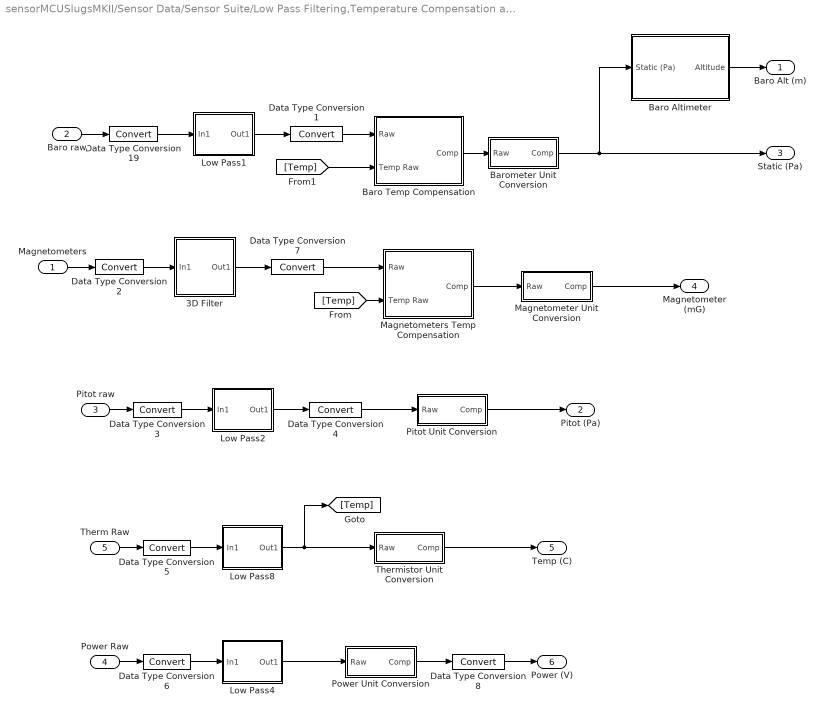
== system sensorMCUSlugsMKII/Sensor Data/Sensor Suite/Low Pass Filtering,Temperature Compensation and Calibration ==
  Magnetometers : Inport
  Baro raw : Inport  Port=2
  Pitot raw : Inport  Port=3
  Power Raw : Inport  Port=4
  Therm Raw : Inport  Port=5
  3D Filter : Subsystem  AncestorBlock=SLUGS_Library/Singnal Routing & Conditioning/3D Filter  RTWFcnName=TustinFilter3D  mask{zval=[], pval=-150, kval=150, TSample=0.01}
      mask prompts: zval "Zeros"; pval "Poles"; kval "Gains"; TSample "Sample Time"
      settings: RTWFcnNameOpts=User specified  RTWFileNameOpts=Use function name
      mask Display:
      | droots(zval,pval,kval)
      | port_label('input',1,'3D')
  Baro Altimeter : Subsystem
  Baro Temp Compensation : Subsystem  mask{alpha=baroTempK, tempMean=baroMeanTemp}
      mask prompts: alpha "Tempearature Coeficient (K_t)"; tempMean "Calibration Temperature Mean (T_avg)"
      mask help:
      | This block implements a temperature compensation. It implmements the following equation:
      |
      | M_tc = M_raw - K_t(T - T_avg)
  Barometer Unit Conversion : Subsystem  mask{bias=baroOffset, gains=baroScale}
      mask prompts: bias "Initial Bias"; gains "Initial Gains"
      mask help: Convert Analog readings to units
  Data Type Conversion1 : DataTypeConversion  OutDataTypeMode=single
  Data Type Conversion{2..3,5..6,19} (5 alike) : DataTypeConversion  OutDataTypeMode=double
  Data Type Conversion4 : DataTypeConversion  OutDataTypeMode=single
  Data Type Conversion7 : DataTypeConversion  OutDataTypeMode=single
  Data Type Conversion8 : DataTypeConversion  OutDataTypeMode=uint16
  Low Pass1 : Subsystem  mask(DiscretizedZeroPole){Zeros=[], Poles=[-30], Gain=30, AbsTol=auto, SampleTime=T, method=tustin, Wc=1}
      mask prompts: Zeros "Zeros (enter in s-main:)"; Poles "Poles (enter in s-domain:)"; Gain "Gain (enter in s-domain:)"; AbsTol "Absolute tolerance:"; SampleTime "Sample time:"; Wc "Critical Frequency (Hz):"
      mask help: Continuous mask uses c2d to transform parameters onto the Discrete Zero-Pole block inside.
      mask init:
      | st=SampleTime;
      | if length(st)>1
      |     st=SampleTime(1);
      | end
      | if(st>0)
      |     [zerosd,polesd,gaind] = sldiscutil('disczpk', {st,method,Wc,Zeros,Poles,Gain});
      | end	
      | s = get_param(gcb,'maskvalues');
      | zeross = s{1};
      | poless = s{2};
      | gainss = s{3};
      | %zerosc = eval(zeross);
      | %polesc = eval(poless);
      | %gainsc = eval(gainss);
      | sldiscutil('initzpkmask', st);
      | if(st==0)
      | set_param([gcb '/Zero Pole'], 'AbsoluteTolerance', AbsTol);
      | end
      mask StyleString: edit,edit,edit,edit,edit,popup(zoh|foh|tustin|prewarp|matched),edit
      mask CallbackString: |||||hidecrit|
      mask Display:
      | droots(zeross,poless,gainss)
      | text( 0.5, 1.0, method, 'verticalAlignment','top')
  Low Pass2 : Subsystem  mask(DiscretizedZeroPole){Zeros=[], Poles=[-30], Gain=30, AbsTol=auto, SampleTime=T, method=tustin, Wc=1}
      mask prompts: Zeros "Zeros (enter in s-main:)"; Poles "Poles (enter in s-domain:)"; Gain "Gain (enter in s-domain:)"; AbsTol "Absolute tolerance:"; SampleTime "Sample time:"; Wc "Critical Frequency (Hz):"
      mask help: Continuous mask uses c2d to transform parameters onto the Discrete Zero-Pole block inside.
      mask init: same as sensorMCUSlugsMKII/Sensor Data/Sensor Suite/Low Pass Filtering,Temperature Compensation and Calibration/Low Pass1
      mask StyleString: edit,edit,edit,edit,edit,popup(zoh|foh|tustin|prewarp|matched),edit
      mask CallbackString: |||||hidecrit|
      mask Display:
      | droots(zeross,poless,gainss)
      | text( 0.5, 1.0, method, 'verticalAlignment','top')
  Low Pass4 : Subsystem  mask(DiscretizedZeroPole){Zeros=[], Poles=[-3], Gain=3, AbsTol=auto, SampleTime=T, method=tustin, Wc=1}
      mask prompts: Zeros "Zeros (enter in s-main:)"; Poles "Poles (enter in s-domain:)"; Gain "Gain (enter in s-domain:)"; AbsTol "Absolute tolerance:"; SampleTime "Sample time:"; Wc "Critical Frequency (Hz):"
      mask help: Continuous mask uses c2d to transform parameters onto the Discrete Zero-Pole block inside.
      mask init: same as sensorMCUSlugsMKII/Sensor Data/Sensor Suite/Low Pass Filtering,Temperature Compensation and Calibration/Low Pass1
      mask StyleString: edit,edit,edit,edit,edit,popup(zoh|foh|tustin|prewarp|matched),edit
      mask CallbackString: |||||hidecrit|
      mask Display:
      | droots(zeross,poless,gainss)
      | text( 0.5, 1.0, method, 'verticalAlignment','top')
  Low Pass8 : Subsystem  mask(DiscretizedZeroPole){Zeros=[], Poles=[-10], Gain=10, AbsTol=auto, SampleTime=T, method=tustin, Wc=1}
      mask prompts: Zeros "Zeros (enter in s-main:)"; Poles "Poles (enter in s-domain:)"; Gain "Gain (enter in s-domain:)"; AbsTol "Absolute tolerance:"; SampleTime "Sample time:"; Wc "Critical Frequency (Hz):"
      mask help: Continuous mask uses c2d to transform parameters onto the Discrete Zero-Pole block inside.
      mask init: same as sensorMCUSlugsMKII/Sensor Data/Sensor Suite/Low Pass Filtering,Temperature Compensation and Calibration/Low Pass1
      mask StyleString: edit,edit,edit,edit,edit,popup(zoh|foh|tustin|prewarp|matched),edit
      mask CallbackString: |||||hidecrit|
      mask Display:
      | droots(zeross,poless,gainss)
      | text( 0.5, 1.0, method, 'verticalAlignment','top')
  Magnetometer Unit Conversion : Subsystem  mask{bias=magOffset, gains=magScale}
      mask prompts: bias "Initial Bias"; gains "Initial Gains"
      mask help: Convert Analog readings to units
  Magnetometers Temp Compensation : Subsystem  mask{alpha=magTempK, tempMean=magMeanTemp}
      mask prompts: alpha "Tempearature Coeficient (K_t)"; tempMean "Calibration Temperature Mean (T_avg)"
      mask help:
      | This block implements a temperature compensation. It implmements the following equation:
      |
      | M_tc = M_raw - K_t(T - T_avg)
  Pitot Unit Conversion : Subsystem  mask{bias=pitotOffset, gains=pitotScale}
      mask prompts: bias "Initial Bias"; gains "Initial Gains"
      mask help: Convert Analog readings to units
  Power Unit Conversion : Subsystem  mask{bias=powerOffset, gains=powerScale}
      mask prompts: bias "Initial Bias"; gains "Initial Gains"
      mask help: Convert Analog readings to units
  Thermistor Unit Conversion : Subsystem  mask{bias=tempOffset, gains=tempScale}
      mask prompts: bias "Initial Bias"; gains "Initial Gains"
      mask help: Convert Analog readings to units
  Baro Alt (m) : Outport
  Pitot (Pa) : Outport  Port=2
  Static (Pa) : Outport  Port=3
  Magnetometer (mG) : Outport  Port=4
  Temp (C) : Outport  Port=5
  Power (V) : Outport  Port=6
  wires:
  Data Type Conversion19/1 -> Low Pass1/1(In1)
  Data Type Conversion3/1 -> Low Pass2/1(In1)
  Low Pass2/1(Out1) -> Data Type Conversion4/1
  Data Type Conversion5/1 -> Low Pass8/1(In1)
  Barometer Unit Conversion/1(Comp) -> Static (Pa)/1, Baro Altimeter/1(Static (Pa))
  Baro raw/1 -> Data Type Conversion19/1
  Pitot raw/1 -> Data Type Conversion3/1
  Therm Raw/1 -> Data Type Conversion5/1
  Baro Temp Compensation/1(Comp) -> Barometer Unit Conversion/1(Raw)
  Data Type Conversion2/1 -> 3D Filter/1(In1)
  3D Filter/1(Out1) -> Data Type Conversion7/1
  Magnetometers/1 -> Data Type Conversion2/1
  Pitot Unit Conversion/1(Comp) -> Pitot (Pa)/1
  Low Pass8/1(Out1) -> [Temp], Thermistor Unit Conversion/1(Raw)
  Data Type Conversion4/1 -> Pitot Unit Conversion/1(Raw)
  Data Type Conversion7/1 -> Magnetometers Temp Compensation/1(Raw)
  Magnetometers Temp Compensation/1(Comp) -> Magnetometer Unit Conversion/1(Raw)
  [Temp] -> Magnetometers Temp Compensation/2(Temp Raw)
  Magnetometer Unit Conversion/1(Comp) -> Magnetometer (mG)/1
  Low Pass1/1(Out1) -> Data Type Conversion1/1
  [Temp] -> Baro Temp Compensation/2(Temp Raw)
  Data Type Conversion1/1 -> Baro Temp Compensation/1(Raw)
  Thermistor Unit Conversion/1(Comp) -> Temp (C)/1
  Data Type Conversion6/1 -> Low Pass4/1(In1)
  Power Raw/1 -> Data Type Conversion6/1
  Low Pass4/1(Out1) -> Power Unit Conversion/1(Raw)
  Power Unit Conversion/1(Comp) -> Data Type Conversion8/1
  Data Type Conversion8/1 -> Power (V)/1
  Baro Altimeter/1(Altitude) -> Baro Alt (m)/1

== system sensorMCUSlugsMKII/Sensor Data/Sensor Suite/Low Pass Filtering,Temperature Compensation and Calibration/3D Filter ==
  In1 : Inport
  Demux : Demux  Outputs=3
  Filter1 : Subsystem  mask(DiscretizedZeroPole){Zeros=zval, Poles=pval, Gain=kval, AbsTol=auto, SampleTime=TSample, method=tustin, Wc=1}
      mask prompts: Zeros "Zeros (enter in s-main:)"; Poles "Poles (enter in s-domain:)"; Gain "Gain (enter in s-domain:)"; AbsTol "Absolute tolerance:"; SampleTime "Sample time:"; Wc "Critical Frequency (Hz):"
      mask help: Continuous mask uses c2d to transform parameters onto the Discrete Zero-Pole block inside.
      mask init: same as sensorMCUSlugsMKII/Sensor Data/Sensor Suite/Low Pass Filtering,Temperature Compensation and Calibration/Low Pass1
      mask StyleString: edit,edit,edit,edit,edit,popup(zoh|foh|tustin|prewarp|matched),edit
      mask CallbackString: |||||hidecrit|
      mask Display:
      | droots(zeross,poless,gainss)
      | text( 0.5, 1.0, method, 'verticalAlignment','top')
  Filter2 : Subsystem  mask(DiscretizedZeroPole){Zeros=zval, Poles=pval, Gain=kval, AbsTol=auto, SampleTime=TSample, method=tustin, Wc=1}
      mask prompts: Zeros "Zeros (enter in s-main:)"; Poles "Poles (enter in s-domain:)"; Gain "Gain (enter in s-domain:)"; AbsTol "Absolute tolerance:"; SampleTime "Sample time:"; Wc "Critical Frequency (Hz):"
      mask help: Continuous mask uses c2d to transform parameters onto the Discrete Zero-Pole block inside.
      mask init: same as sensorMCUSlugsMKII/Sensor Data/Sensor Suite/Low Pass Filtering,Temperature Compensation and Calibration/Low Pass1
      mask StyleString: edit,edit,edit,edit,edit,popup(zoh|foh|tustin|prewarp|matched),edit
      mask CallbackString: |||||hidecrit|
      mask Display:
      | droots(zeross,poless,gainss)
      | text( 0.5, 1.0, method, 'verticalAlignment','top')
  Filter3 : Subsystem  mask(DiscretizedZeroPole){Zeros=zval, Poles=pval, Gain=kval, AbsTol=auto, SampleTime=TSample, method=tustin, Wc=1}
      mask prompts: Zeros "Zeros (enter in s-main:)"; Poles "Poles (enter in s-domain:)"; Gain "Gain (enter in s-domain:)"; AbsTol "Absolute tolerance:"; SampleTime "Sample time:"; Wc "Critical Frequency (Hz):"
      mask help: Continuous mask uses c2d to transform parameters onto the Discrete Zero-Pole block inside.
      mask init: same as sensorMCUSlugsMKII/Sensor Data/Sensor Suite/Low Pass Filtering,Temperature Compensation and Calibration/Low Pass1
      mask StyleString: edit,edit,edit,edit,edit,popup(zoh|foh|tustin|prewarp|matched),edit
      mask CallbackString: |||||hidecrit|
      mask Display:
      | droots(zeross,poless,gainss)
      | text( 0.5, 1.0, method, 'verticalAlignment','top')
  myMux Fun1 : Stateflow chart
  Out1 : Outport
  wires:
  myMux Fun1/1(y) -> Out1/1
  In1/1 -> Demux/1
  Filter3/1(Out1) -> myMux Fun1/3(u3)
  Filter2/1(Out1) -> myMux Fun1/2(u2)
  Filter1/1(Out1) -> myMux Fun1/1(u1)
  Demux/3 -> Filter3/1(In1)
  Demux/2 -> Filter2/1(In1)
  Demux/1 -> Filter1/1(In1)

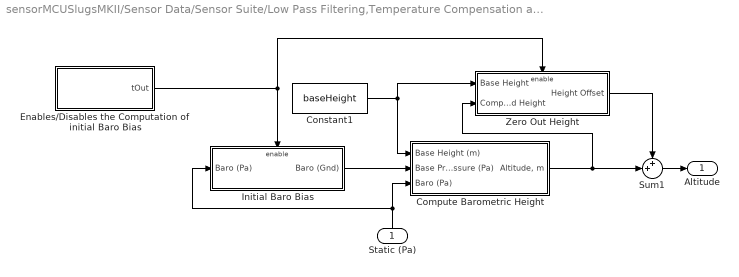
== system sensorMCUSlugsMKII/Sensor Data/Sensor Suite/Low Pass Filtering,Temperature Compensation and Calibration/Baro Altimeter ==
  Static (Pa) : Inport  Orientation=up
  Compute Barometric Height : Subsystem  mask{baseTemp=baseTemp, LapseRate=lapseRate}
      mask prompts: baseTemp "Base Station Temperature (K)"; LapseRate "Lapse Rate (C/ft)"
      mask help:
      | Produces Altitude in meters from Barometric Pressure in Pascals. Altitude is valid from MSL to 6000 ft.
      |
      | The method implemented here was developed by Ren Curry
  Constant1 : Constant  Value=baseHeight  OutDataTypeMode=single
  Enables/Disables the Computation of  initial Baro Bias : Stateflow chart
  Initial Baro Bias : Subsystem  TreatAsAtomicUnit=on
  Sum1 : Sum  Inputs=++|  OutDataTypeMode=single
  Zero Out Height : Subsystem  TreatAsAtomicUnit=on
  Altitude : Outport
  wires:
  Compute Barometric Height/1("Altitude, m") -> Zero Out Height/2(Computed Height), Sum1/2
  Static (Pa)/1 -> Initial Baro Bias/1(Baro (Pa)), Compute Barometric Height/3(Baro (Pa))
  Enables/Disables the Computation of  initial Baro Bias/1(tOut) -> Initial Baro Bias/Enable, Zero Out Height/Enable
  Constant1/1 -> Compute Barometric Height/1(Base Height (m)), Zero Out Height/1(Base Height)
  Initial Baro Bias/1(Baro (Gnd)) -> Compute Barometric Height/2(Base Pressure (Pa))
  Zero Out Height/1(Height Offset) -> Sum1/1
  Sum1/1 -> Altitude/1

== system sensorMCUSlugsMKII/Sensor Data/Sensor Suite/Low Pass Filtering,Temperature Compensation and Calibration/Baro Temp Compensation ==
  Raw : Inport
  Temp Raw : Inport  Port=2
  Divide1 : Product  OutDataTypeMode=single  OutScaling=2^-10
  Mean Temperature for Calibration : Constant  Value=tempMean  OutDataTypeMode=single
  Sum1 : Sum  Inputs=|+-  OutDataTypeMode=single
  Sum2 : Sum  Inputs=|+-  OutDataTypeMode=single
  gains : Constant  Value=alpha  OutDataTypeMode=single
  Comp : Outport
  wires:
  Mean Temperature for Calibration/1 -> Sum1/2
  Raw/1 -> Sum2/1
  Temp Raw/1 -> Sum1/1
  Sum1/1 -> Divide1/2
  gains/1 -> Divide1/1
  Divide1/1 -> Sum2/2
  Sum2/1 -> Comp/1

== system sensorMCUSlugsMKII/Sensor Data/Sensor Suite/Low Pass Filtering,Temperature Compensation and Calibration/Barometer Unit Conversion ==
  Raw : Inport
  Bias : Constant  Value=bias  OutDataTypeMode=single
  Divide : Product  OutDataTypeMode=single  OutScaling=2^-10
  Gains : Constant  Value=gains  OutDataTypeMode=single
  Sum : Sum  Inputs=|++  OutDataTypeMode=single
  Comp : Outport
  wires:
  Bias/1 -> Sum/2
  Raw/1 -> Divide/2
  Gains/1 -> Divide/1
  Divide/1 -> Sum/1
  Sum/1 -> Comp/1

== system sensorMCUSlugsMKII/Sensor Data/Sensor Suite/Low Pass Filtering,Temperature Compensation and Calibration/Low Pass1 ==
  In1 : Inport
  Discrete Zero-Pole : DiscreteZeroPole  Zeros=zerosd  Poles=polesd  Gain=gaind  SampleTime=SampleTime
  Out1 : Outport
  wires:
  In1/1 -> Discrete Zero-Pole/1
  Discrete Zero-Pole/1 -> Out1/1

== system sensorMCUSlugsMKII/Sensor Data/Sensor Suite/Low Pass Filtering,Temperature Compensation and Calibration/Low Pass2 ==
  In1 : Inport
  Discrete Zero-Pole : DiscreteZeroPole  Zeros=zerosd  Poles=polesd  Gain=gaind  SampleTime=SampleTime
  Out1 : Outport
  wires:
  Discrete Zero-Pole/1 -> Out1/1
  In1/1 -> Discrete Zero-Pole/1

== system sensorMCUSlugsMKII/Sensor Data/Sensor Suite/Low Pass Filtering,Temperature Compensation and Calibration/Low Pass4 ==
  In1 : Inport
  Discrete Zero-Pole : DiscreteZeroPole  Zeros=zerosd  Poles=polesd  Gain=gaind  SampleTime=SampleTime
  Out1 : Outport
  wires:
  Discrete Zero-Pole/1 -> Out1/1
  In1/1 -> Discrete Zero-Pole/1

== system sensorMCUSlugsMKII/Sensor Data/Sensor Suite/Low Pass Filtering,Temperature Compensation and Calibration/Low Pass8 ==
  In1 : Inport
  Discrete Zero-Pole : DiscreteZeroPole  Zeros=zerosd  Poles=polesd  Gain=gaind  SampleTime=SampleTime
  Out1 : Outport
  wires:
  In1/1 -> Discrete Zero-Pole/1
  Discrete Zero-Pole/1 -> Out1/1

== system sensorMCUSlugsMKII/Sensor Data/Sensor Suite/Low Pass Filtering,Temperature Compensation and Calibration/Magnetometer Unit Conversion ==
  Raw : Inport
  Bias : Constant  Value=bias  OutDataTypeMode=single
  Divide : Product  OutDataTypeMode=single  OutScaling=2^-10
  Gains : Constant  Value=gains  OutDataTypeMode=single
  Sum : Sum  Inputs=|++  OutDataTypeMode=single
  Comp : Outport
  wires:
  Sum/1 -> Comp/1
  Divide/1 -> Sum/1
  Gains/1 -> Divide/1
  Raw/1 -> Divide/2
  Bias/1 -> Sum/2

== system sensorMCUSlugsMKII/Sensor Data/Sensor Suite/Low Pass Filtering,Temperature Compensation and Calibration/Magnetometers Temp Compensation ==
  Raw : Inport
  Temp Raw : Inport  Port=2
  Divide1 : Product  OutDataTypeMode=single  OutScaling=2^-10
  Mean Temperature for Calibration : Constant  Value=tempMean  OutDataTypeMode=single
  Sum1 : Sum  Inputs=|+-  OutDataTypeMode=single
  Sum2 : Sum  Inputs=|+-  OutDataTypeMode=single
  gains : Constant  Value=alpha  OutDataTypeMode=single
  Comp : Outport
  wires:
  Sum2/1 -> Comp/1
  Divide1/1 -> Sum2/2
  gains/1 -> Divide1/1
  Sum1/1 -> Divide1/2
  Temp Raw/1 -> Sum1/1
  Raw/1 -> Sum2/1
  Mean Temperature for Calibration/1 -> Sum1/2

== system sensorMCUSlugsMKII/Sensor Data/Sensor Suite/Low Pass Filtering,Temperature Compensation and Calibration/Pitot Unit Conversion ==
  Raw : Inport
  Bias : Constant  Value=bias  OutDataTypeMode=single
  Divide : Product  OutDataTypeMode=single  OutScaling=2^-10
  Gains : Constant  Value=gains  OutDataTypeMode=single
  Sum : Sum  Inputs=|++  OutDataTypeMode=single
  Comp : Outport
  wires:
  Bias/1 -> Sum/2
  Raw/1 -> Divide/2
  Gains/1 -> Divide/1
  Divide/1 -> Sum/1
  Sum/1 -> Comp/1

== system sensorMCUSlugsMKII/Sensor Data/Sensor Suite/Low Pass Filtering,Temperature Compensation and Calibration/Power Unit Conversion ==
  Raw : Inport
  Bias : Constant  Value=bias  OutDataTypeMode=single
  Divide : Product  OutDataTypeMode=single  OutScaling=2^-10
  Gains : Constant  Value=gains  OutDataTypeMode=single
  Sum : Sum  Inputs=|++  OutDataTypeMode=single
  Comp : Outport
  wires:
  Bias/1 -> Sum/2
  Raw/1 -> Divide/2
  Gains/1 -> Divide/1
  Divide/1 -> Sum/1
  Sum/1 -> Comp/1

== system sensorMCUSlugsMKII/Sensor Data/Sensor Suite/Low Pass Filtering,Temperature Compensation and Calibration/Thermistor Unit Conversion ==
  Raw : Inport
  Bias : Constant  Value=bias  OutDataTypeMode=single
  Divide : Product  OutDataTypeMode=single  OutScaling=2^-10
  Gains : Constant  Value=gains  OutDataTypeMode=single
  Sum : Sum  Inputs=|++  OutDataTypeMode=single
  Comp : Outport
  wires:
  Sum/1 -> Comp/1
  Divide/1 -> Sum/1
  Gains/1 -> Divide/1
  Raw/1 -> Divide/2
  Bias/1 -> Sum/2

== system sensorMCUSlugsMKII/Sensor Data/Sensor Suite/Low Pass Filtering,Temperature Compensation and Calibration/3D Filter/Filter1 ==
  In1 : Inport
  Discrete Zero-Pole : DiscreteZeroPole  Zeros=zerosd  Poles=polesd  Gain=gaind  SampleTime=SampleTime
  Out1 : Outport
  wires:
  Discrete Zero-Pole/1 -> Out1/1
  In1/1 -> Discrete Zero-Pole/1

== system sensorMCUSlugsMKII/Sensor Data/Sensor Suite/Low Pass Filtering,Temperature Compensation and Calibration/3D Filter/Filter2 ==
  In1 : Inport
  Discrete Zero-Pole : DiscreteZeroPole  Zeros=zerosd  Poles=polesd  Gain=gaind  SampleTime=SampleTime
  Out1 : Outport
  wires:
  In1/1 -> Discrete Zero-Pole/1
  Discrete Zero-Pole/1 -> Out1/1

== system sensorMCUSlugsMKII/Sensor Data/Sensor Suite/Low Pass Filtering,Temperature Compensation and Calibration/3D Filter/Filter3 ==
  In1 : Inport
  Discrete Zero-Pole : DiscreteZeroPole  Zeros=zerosd  Poles=polesd  Gain=gaind  SampleTime=SampleTime
  Out1 : Outport
  wires:
  Discrete Zero-Pole/1 -> Out1/1
  In1/1 -> Discrete Zero-Pole/1

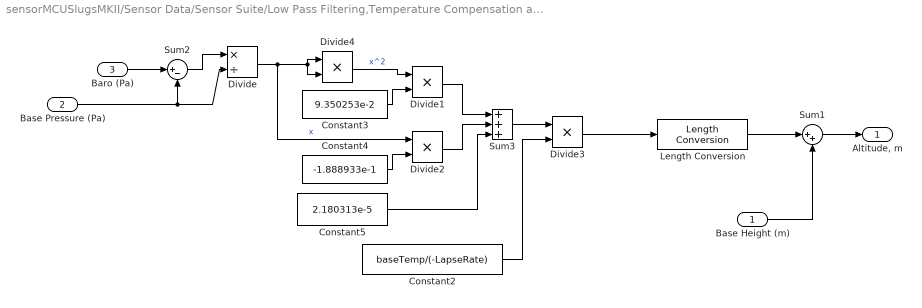
== system sensorMCUSlugsMKII/Sensor Data/Sensor Suite/Low Pass Filtering,Temperature Compensation and Calibration/Baro Altimeter/Compute Barometric Height ==
  Base Height (m) : Inport
  Base Pressure (Pa) : Inport  Port=2
  Baro (Pa) : Inport  Port=3
  Constant2 : Constant  Value=baseTemp/(-LapseRate)  OutDataTypeMode=single
  Constant3 : Constant  Value=9.350253e-2  OutDataTypeMode=single
  Constant4 : Constant  Value=-1.888933e-1  OutDataTypeMode=single
  Constant5 : Constant  Value=2.180313e-5  OutDataTypeMode=single
  Divide : Product  Inputs=*/  OutDataTypeMode=single  OutScaling=2^-10
  Divide{1..4} (4 alike) : Product  OutDataTypeMode=single  OutScaling=2^-10
  Length Conversion : aerolibconvert2/Length Conversion  SystemSampleTime=-1  IU=ft  OU=m
  Sum1 : Sum  Inputs=|++  OutDataTypeMode=single
  Sum2 : Sum  Inputs=|+-  OutDataTypeMode=single
  Sum3 : Sum  Inputs=3  OutDataTypeMode=single
  "Altitude, m" : Outport
  wires:
  Length Conversion/1 -> Sum1/1
  Sum2/1 -> Divide/1
  Sum1/1 -> "Altitude, m"/1
  Divide3/1 -> Length Conversion/1
  Constant2/1 -> Divide3/2
  Sum3/1 -> Divide3/1
  Constant5/1 -> Sum3/3
  Divide2/1 -> Sum3/2
  Divide1/1 -> Sum3/1
  Constant4/1 -> Divide2/2
  Constant3/1 -> Divide1/2
  Divide4/1 -> Divide1/1  "x^2"
  Divide/1 -> Divide2/1, Divide4/1, Divide4/2  "x"
  Base Pressure (Pa)/1 -> Divide/2, Sum2/2
  Base Height (m)/1 -> Sum1/2
  Baro (Pa)/1 -> Sum2/1
